simulink library "AtmosferModel"  (R2023a)
settings: Solver=VariableStepAuto  StartTime=0.0  StopTime=10.0  RelTol=1e-3
settings Model: Creator=User  LastModifiedBy=User

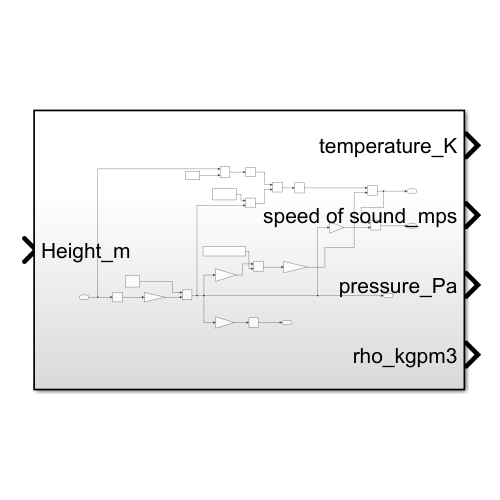
[thumbnail: Simulink's stored preview of the top-level diagram]
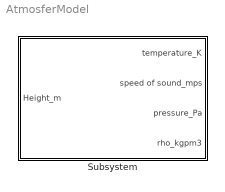
== system AtmosferModel ==
  Subsystem : Subsystem

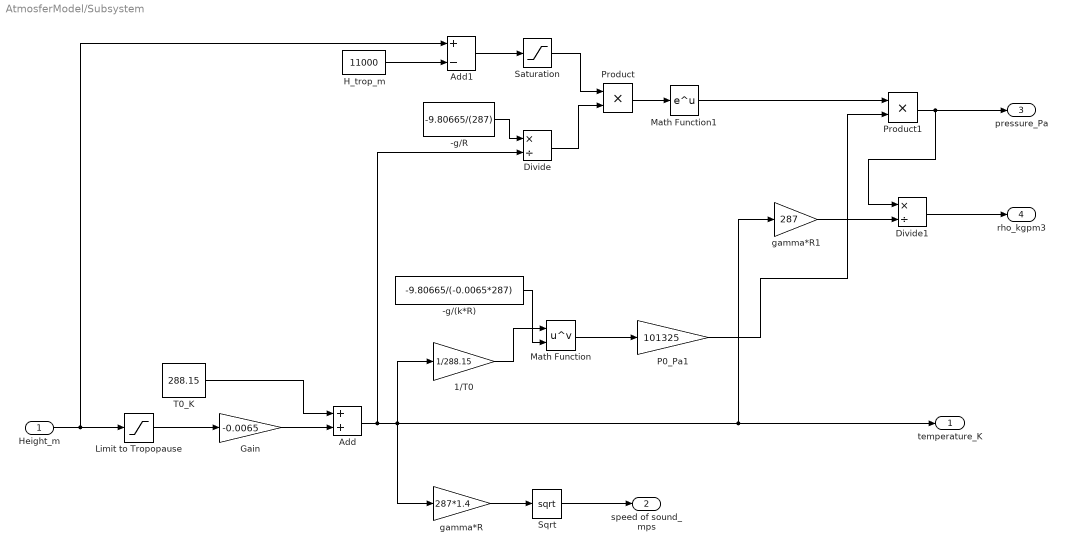
== system AtmosferModel/Subsystem ==
  Height_m : Inport
  -g/(k*R) : Constant  Value=-9.80665/(-0.0065*287)
  -g/R : Constant  Value=-9.80665/(287)
  1/T0 : Gain  Gain=1/288.15
  Add : Sum
  Add1 : Sum  Inputs=+-
  Divide : Product  Inputs=*/
  Divide1 : Product  Inputs=*/
  Gain : Gain  Gain=-0.0065
  H_trop_m : Constant  Value=11000
  Limit to Tropopause : Saturate  UpperLimit=1100  LowerLimit=0
  Math Function : Math  Operator=pow
  Math Function1 : Math
  P0_Pa1 : Gain  Gain=101325
  Product : Product
  Product1 : Product
  Saturation : Saturate  UpperLimit=inf  LowerLimit=0
  Sqrt : Sqrt
  T0_K : Constant  Value=288.15
  gamma*R : Gain  Gain=287*1.4
  gamma*R1 : Gain  Gain=287
  temperature_K : Outport
  speed of sound_mps : Outport  Port=2
  pressure_Pa : Outport  Port=3
  rho_kgpm3 : Outport  Port=4
  wires:
  gamma*R/1 -> Sqrt/1
  Saturation/1 -> Product/1
  Math Function1/1 -> Product1/1
  Add/1 -> Divide/2, 1/T0/1, gamma*R/1, temperature_K/1, gamma*R1/1
  T0_K/1 -> Add/1
  Height_m/1 -> Add1/1, Limit to Tropopause/1
  Math Function/1 -> P0_Pa1/1
  Product1/1 -> pressure_Pa/1, Divide1/1
  Gain/1 -> Add/2
  Add1/1 -> Saturation/1
  -g/(k*R)/1 -> Math Function/2
  gamma*R1/1 -> Divide1/2
  P0_Pa1/1 -> Product1/2
  Divide1/1 -> rho_kgpm3/1
  1/T0/1 -> Math Function/1
  Product/1 -> Math Function1/1
  -g/R/1 -> Divide/1
  H_trop_m/1 -> Add1/2
  Limit to Tropopause/1 -> Gain/1
  Divide/1 -> Product/2
  Sqrt/1 -> speed of sound_mps/1
